simulink model "USV1_Trajectory_Simulink"  (R2018a)
settings: Solver=VariableStepAuto  StartTime=0.0  StopTime=200  RelTol=1e-3
values from neighbouring files (symbols this model uses):
  A = [A_CAME; A_IKE; A_CLME]    [Prototype.m]    (also in USV1_PID_Fuzzy_Parameters.m = Mass\(-Coriolis - D_l))
  B = [B_CAME; B_IKE; B_CLME]    [Prototype.m]    (also in USV1_PID_Fuzzy_Parameters.m = Mass\F)
  C = eye(9)    [Prototype.m]    (also in USV1_PID_Fuzzy_Parameters.m = eye(4))
  Condition = [0;0;0;0.1;0.1;0;0;0;0]    [Prototype.m]    (also in USV1_PID_Fuzzy_Parameters.m = [1; 0; 0; 3*pi/4])
  D = zeros(9,4)    [Prototype.m]    (also in USV1_PID_Fuzzy_Parameters.m = [ 0  0  0 ;       0  0  0 ;       0  0  0 ;       0  0  0 ])
  Width = 1.83    [USV1_PID_Fuzzy_Parameters.m]
settings Model: Creator=admin  LastModifiedBy=admin

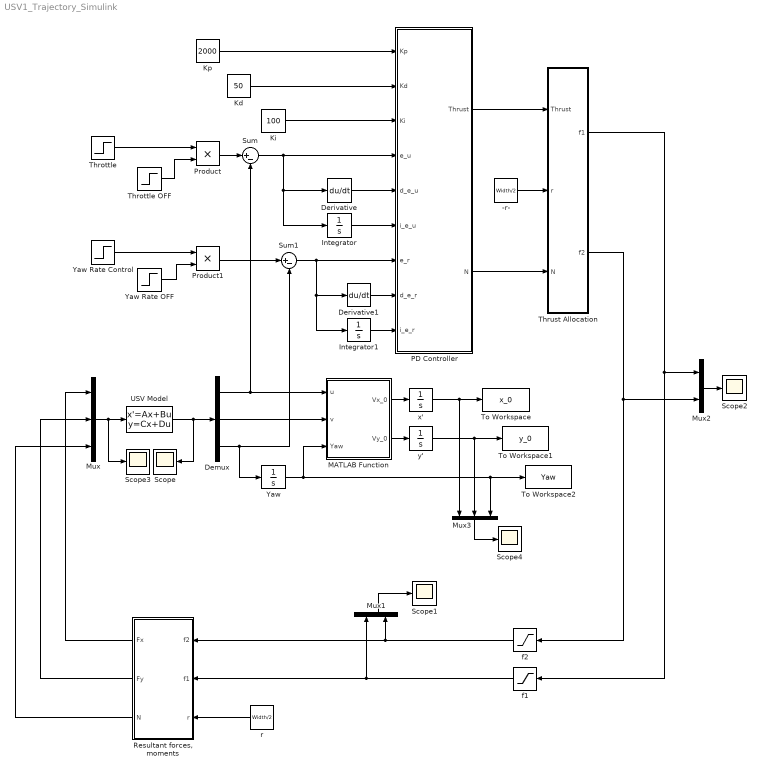
== system USV1_Trajectory_Simulink ==
  "-r- " : Constant  Value=Width/2
  Demux : Demux  Outputs=3
  Derivative : Derivative
  Derivative1 : Derivative
  Integrator : Integrator
  Integrator1 : Integrator
  "Kd " : Constant  Value=50
  Ki : Constant  Value=100
  Kp : Constant  Value=2000
  MATLAB Function : MATLAB Function  TreatAsAtomicUnit=on
  Mux : Mux  Inputs=3
  Mux1 : Mux  Inputs=2
  Mux2 : Mux  Inputs=2
  Mux3 : Mux  Inputs=3
  PD Controller : MATLAB Function  TreatAsAtomicUnit=on
  Product : Product
  Product1 : Product
  "Resultant forces, moments" : MATLAB Function  TreatAsAtomicUnit=on
  Scope{,1..4} (5 alike) : Scope
  Sum : Sum  Inputs=|+-
  Sum1 : Sum  Inputs=|+-
  Throttle : Step  After=0.9  SampleTime=10
  Throttle OFF : Step  Before=1  SampleTime=30
  Thrust Allocation : MATLAB Function  TreatAsAtomicUnit=on
  To Workspace : ToWorkspace  VariableName=x_0  SampleTime=-1
  To Workspace1 : ToWorkspace  VariableName=y_0  SampleTime=-1
  To Workspace2 : ToWorkspace  VariableName=Yaw  SampleTime=-1
  USV Model : StateSpace  A=A  B=B  C=C  D=D  InitialCondition=Condition
  Yaw : Integrator
  Yaw Rate OFF : Step  Before=1  After=0  SampleTime=80
  Yaw Rate Control : Step  After=0.17  SampleTime=60
  f1 : Saturate  UpperLimit=100  LowerLimit=0
  f2 : Saturate  UpperLimit=100  LowerLimit=0
  r : Constant  Value=Width/2
  x' : Integrator
  y' : Integrator
  wires:
  USV Model/1 -> Scope/1, Demux/1
  Mux/1 -> Scope3/1, USV Model/1
  Demux/1 -> MATLAB Function/1(u), Sum/2
  Product1/1 -> Sum1/1
  Demux/3 -> Yaw/1, Sum1/2
  Sum/1 -> Integrator/1, Derivative/1, PD Controller/4(e_u)
  Sum1/1 -> Integrator1/1, Derivative1/1, PD Controller/7(e_r)
  Derivative/1 -> PD Controller/5(d_e_u)
  Derivative1/1 -> PD Controller/8(d_e_r)
  f1/1 -> "Resultant forces, moments"/2(f1), Mux1/1
  f2/1 -> "Resultant forces, moments"/1(f2), Mux1/2
  r/1 -> "Resultant forces, moments"/3(r)
  "Resultant forces, moments"/1(Fx) -> Mux/1
  "Resultant forces, moments"/2(Fy) -> Mux/2
  "Resultant forces, moments"/3(N) -> Mux/3
  Mux1/1 -> Scope1/1
  "Kd "/1 -> PD Controller/2(Kd)
  Kp/1 -> PD Controller/1(Kp)
  PD Controller/2(N) -> Thrust Allocation/3(N)
  "-r- "/1 -> Thrust Allocation/2(r)
  PD Controller/1(Thrust) -> Thrust Allocation/1(Thrust)
  Thrust Allocation/1(f1) -> Mux2/1, f1/1
  Thrust Allocation/2(f2) -> Mux2/2, f2/1
  Mux2/1 -> Scope2/1
  Throttle/1 -> Product/1
  Throttle OFF/1 -> Product/2
  Product/1 -> Sum/1
  Yaw Rate OFF/1 -> Product1/2
  Yaw Rate Control/1 -> Product1/1
  Ki/1 -> PD Controller/3(Ki)
  Integrator/1 -> PD Controller/6(i_e_u)
  Integrator1/1 -> PD Controller/9(i_e_r)
  Demux/2 -> MATLAB Function/2(v)
  Yaw/1 -> Mux3/3, To Workspace2/1, MATLAB Function/3(Yaw)
  MATLAB Function/1(Vx_0) -> x'/1
  MATLAB Function/2(Vy_0) -> y'/1
  x'/1 -> Mux3/1, To Workspace/1
  y'/1 -> Mux3/2, To Workspace1/1
  Mux3/1 -> Scope4/1

== matlab function USV1_Trajectory_Simulink/Resultant forces, moments ==
  data: f2 input; f1 input; r input; Fx output; Fy output; N output
function [Fx,Fy,N] = fcn(f2,f1,r)

Fx = f1 + f2;
Fy = 0;
N = f1*r - f2*r;

== matlab function USV1_Trajectory_Simulink/PD Controller ==
  data: Kp input; Thrust output; Kd input; Ki input; e_u input; d_e_u input; i_e_u input; e_r input; d_e_r input; N output; i_e_r input
function [Thrust, N] = fcn(Kp, Kd, Ki, e_u,d_e_u,i_e_u, e_r,d_e_r,i_e_r)

Thrust = (e_u * Kp) + (d_e_u * Kd) + (i_e_u * Ki);
N = (e_r * Kp) + (d_e_r * Kd) + (i_e_r * Ki);

== matlab function USV1_Trajectory_Simulink/Thrust Allocation ==
  data: Thrust input; r input; f1 output; N input; f2 output
function [f1,f2] = fcn(Thrust, r, N)

f1 = Thrust/2 + N/r;
f2 = Thrust/2 - N/r;

== matlab function USV1_Trajectory_Simulink/MATLAB Function ==
  data: u input; Vx_0 output; v input; Yaw input; Vy_0 output
function [Vx_0 , Vy_0 ] = fcn(u, v, Yaw)

Vx_0 =  cos(Yaw)*u - sin(Yaw)*v ;
Vy_0 =  sin(Yaw)*u + cos(Yaw)*v ;
